simulink model "uavSim"  (Simulink 7.9)
settings: Solver=ode1  StartTime=0.0  StopTime=100  FixedStep=0.05  RelTol=1e-3
settings Model: Creator=Administrator  LastModifiedBy=Administrator
settings OptimizationCC: InitFltsAndDblsToZero=on
settings DebuggingCC: FcnCallInpInsideContextMsg=Use local settings  StrictBusMsg=Warning
settings GRTTargetCC: CombineOutputUpdateFcns=off  GRTInterface=on

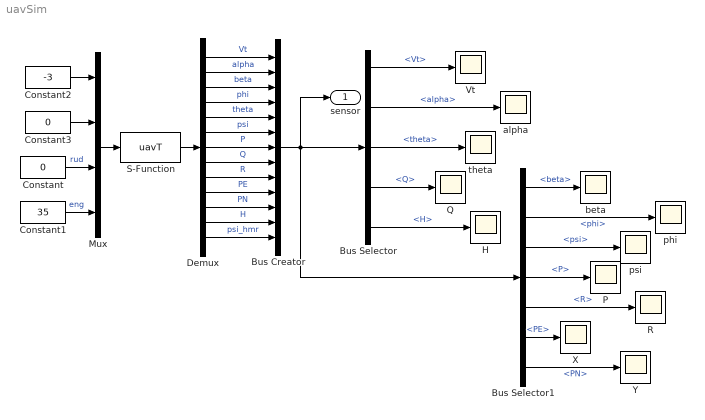
== system uavSim ==
  Bus Creator : BusCreator  Inputs=13
  Bus Selector : BusSelector  OutputSignals=Vt,alpha,theta,Q,H
  Bus Selector1 : BusSelector  OutputSignals=beta,phi,psi,P,R,PE,PN
  Constant : Constant  Value=0
  Constant1 : Constant  Value=35
  Constant2 : Constant  Value=-3
  Constant3 : Constant  Value=0
  Demux : Demux  Outputs=13
  H : Scope
      settings: SaveName=ScopeData4
  Mux : Mux
  P : Scope
      settings: SaveName=ScopeData6
  Q : Scope
      settings: SaveName=ScopeData3
  R : Scope
      settings: SaveName=ScopeData5
  S-Function : S-Function  FunctionName=uavT  EnableBusSupport=off
  Vt : Scope
  X : Scope
      settings: SaveName=ScopeData11
  Y : Scope
      settings: SaveName=ScopeData10
  alpha : Scope
  beta : Scope
      settings: SaveName=ScopeData7
  phi : Scope
      settings: YMin=0.0575  YMax=0.0875  SaveName=ScopeData8
  psi : Scope
      settings: SaveName=ScopeData9
  theta : Scope
      settings: SaveName=ScopeData2
  sensor : Outport
  wires:
  S-Function/1 -> Demux/1
  Demux/1 -> Bus Creator/1  "Vt"
  Demux/2 -> Bus Creator/2  "alpha"
  Demux/3 -> Bus Creator/3  "beta"
  Demux/4 -> Bus Creator/4  "phi"
  Demux/5 -> Bus Creator/5  "theta"
  Demux/6 -> Bus Creator/6  "psi"
  Demux/7 -> Bus Creator/7  "P"
  Demux/8 -> Bus Creator/8  "Q"
  Demux/9 -> Bus Creator/9  "R"
  Demux/10 -> Bus Creator/10  "PE"
  Demux/11 -> Bus Creator/11  "PN"
  Demux/12 -> Bus Creator/12  "H"
  Demux/13 -> Bus Creator/13  "psi_hmr"
  Bus Creator/1 -> sensor/1, Bus Selector/1, Bus Selector1/1
  Bus Selector/1 -> Vt/1  "<Vt>"
  Bus Selector/2 -> alpha/1  "<alpha>"
  Bus Selector/3 -> theta/1  "<theta>"
  Bus Selector/4 -> Q/1  "<Q>"
  Bus Selector/5 -> H/1  "<H>"
  Mux/1 -> S-Function/1
  Constant/1 -> Mux/3  "rud"
  Bus Selector1/1 -> beta/1  "<beta>"
  Bus Selector1/2 -> phi/1  "<phi>"
  Bus Selector1/3 -> psi/1  "<psi>"
  Bus Selector1/4 -> P/1  "<P>"
  Bus Selector1/5 -> R/1  "<R>"
  Bus Selector1/7 -> Y/1  "<PN>"
  Bus Selector1/6 -> X/1  "<PE>"
  Constant1/1 -> Mux/4  "eng"
  Constant2/1 -> Mux/1
  Constant3/1 -> Mux/2
